simulink model "muscle_inputs"  (Simulink 6.4)
settings: Solver=ode45  StartTime=0.0  StopTime=10.0  RelTol=1e-3
settings Model: LastModifiedBy=chadwick

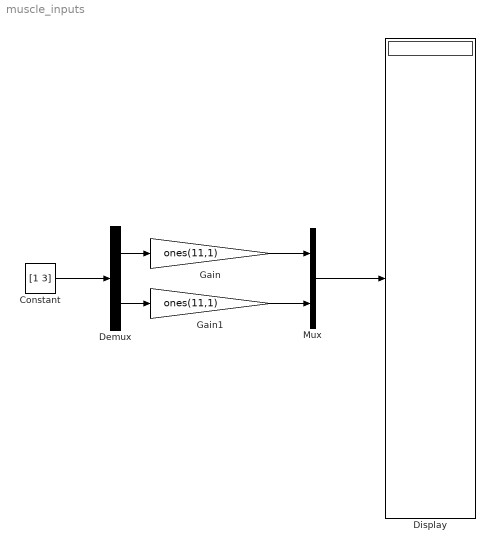
== system muscle_inputs ==
  Constant : Constant  Value=[1 3]  OutDataType=sfix(16)  ConRadixGroup=Use specified scaling  OutScaling=2^0  SampleTime=inf  FramePeriod=inf
  Demux : Demux  Outputs=2
  Display : Display
  Gain : Gain  Gain=ones(11,1)
  Gain1 : Gain  Gain=ones(11,1)
  Mux : Mux  Inputs=2
  wires:
  Demux/1 -> Gain/1
  Demux/2 -> Gain1/1
  Gain/1 -> Mux/1
  Gain1/1 -> Mux/2
  Constant/1 -> Demux/1
  Mux/1 -> Display/1
